simulink model "ROVSim_dp"  (R2022b)
settings: Solver=ode4  StartTime=0.0  StopTime=120  FixedStep=0.05  RelTol=1e-3
InitFcn:
  | initModelParam;
StopFcn:
  | %plotCoupled3DTrack;
libraries: slpidlib x9
settings Model: SimulationMode=accelerator  Creator=53549  LastModifiedBy=18144
settings SolverCC: AlgebraicLoopSolver=TrustRegion
settings DataIOCC: ReturnWorkspaceOutputs=off
settings DebuggingCC: UnconnectedInputMsg=warning  UnconnectedOutputMsg=warning  UnconnectedLineMsg=warning  SFMachineParentedDataDiag=warning  ArithmeticOperatorsInVariantConditions=warning
settings ModelReferenceCC: EnableRefExpFcnMdlSchedulingChecks=on
settings SFSimCC: SimUseLocalCustomCode=off  CustomCodeUndefinedFunction=UseInterfaceOnly
settings RTWCC: RTWUseLocalCustomCode=off  DLArmComputeVersion=19.05
settings CodeAppCC: StateflowObjectComments=on

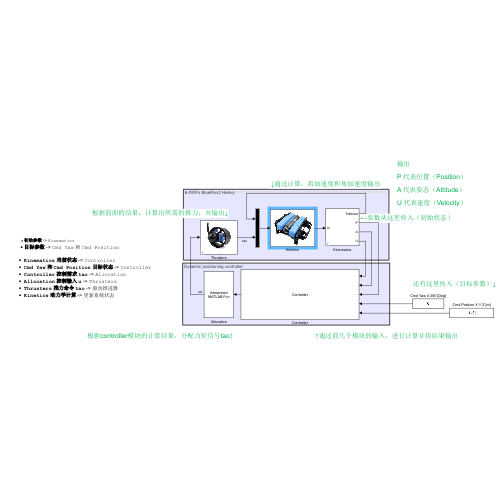
[thumbnail: Simulink's stored preview of the top-level diagram]
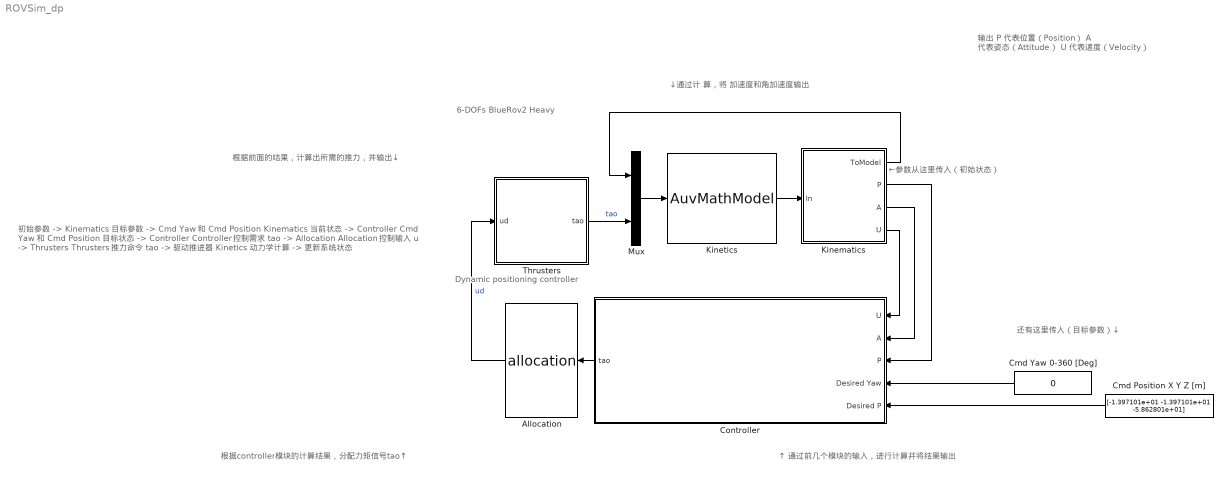
== system ROVSim_dp ==
  note: 初始参数 -> Kinematics
      | 目标参数 -> Cmd Yaw 和 Cmd Position
      |
      | Kinematics 当前状态 -> Controller
      | Cmd Yaw 和 Cmd Position 目标状态 -> Controller
      | Controller 控制需求 tao -> Allocation
      | Allocation 控制输入 u -> Thrusters
      | Thrusters 推力命令 tao -> 驱动推进器
      | Kinetics 动力学计算 -> 更新系统状态
  note: 输出
      | P 代表位置（Position）
      | A 代表姿态（Attitude）
      | U 代表速度（Velocity）
  note: ←参数从这里传入（初始状态）
  note: Dynamic positioning controller
  note: 6-DOFs BlueRov2 Heavy
  note: 还有这里传入（目标参数）↓
  note: ↑ 通过前几个模块的输入，进行计算并将结果输出
  note: 根据controller模块的计算结果，分配力矩信号tao↑
  note: 根据前面的结果，计算出所需的推力，并输出↓
  note: ↓通过计 算，将 加速度和角加速度输出
  Allocation : MATLABFcn  Description=|  MATLABFcn=allocation  OutputDimensions=8  OutputSignalType=real
      | Allocation模块功能:
      |  - 接收控制力和力矩信号tao
      |  - 使用控制分配矩阵Kni和转换矩阵Tni
      |  - 通过矩阵乘法将控制需求分配到各个推进器或执行机构
      |  - 输出控制输入u，用于驱动推进器或其他执行机构
  Cmd Position X Y Z [m] : Constant  Value=[-1.397101e+01 -1.397101e+01 -5.862801e+01]
  Cmd Yaw 0-360 [Deg] : Constant  Value=0
  Controller : Subsystem  Description=|
      | Controller模块功能:
      |  - 接收当前的位置信号P和姿态信号A
      |  - 接收期望的目标位置Desired P和艏向Desired Yaw
      |  - 通过PID控制器计算各个方向和角度的控制力和力矩信号
      |  - 输出控制信号tao_X、tao_Y、tao_Z、tao_K、tao_M和tao_N
      |  - 这些控制信号用于驱动船只的推进器或其他执行机构
      |  - 实现船只的精确运动和姿态控制
      mask Display: disp('Controller')
  Kinematics : Subsystem  Description=|  mask{x0=0.00, y0=0.00, z0=-40.00, pitch0=0, yaw0=138.72, u0=0, flowDir=45, flowVel=0.2}
      | 模块结构分析
      | 输入信号：
      | 包括线速度（u, v, w）和角速度（p, q, r）的信号，这些信号来自于动力学模块或其他部分。
      | 积分运算：
      | 通过积分角速度得到姿态角度，通过积分线速度得到位置坐标。
      | 输出信号：
      | 输出位置（P）、姿态（A）和速度（U），这些信号被其他模块使用，例如控制器、导航系统等。
      mask prompts: x0 "Initiral x"; y0 "Initiral y"; z0 "Initiral z"; pitch0 "Initial pitch [Deg]"; yaw0 "Initial yaw [Deg]"; u0 "Initial velocity [m/s]"; flowDir "Flow direction [Deg]"; flowVel "Flow velocity [m/s]"
      mask DialogControl DescGroupVar Prompt: Kinematics
      mask DialogControl DescTextVar Prompt: Set kinematics information: AMV initial state, flow interference, etc
      mask DialogControl ParameterGroupVar Prompt: Initial state
      mask DialogControl Container3 Prompt: Flow
  Kinetics : MATLABFcn  Description=|  MATLABFcn=AuvMathModel  OutputDimensions=6  OutputSignalType=real
      | Kinetics模块功能:
      |  - 接收当前的速度、角速度、姿态角度和控制力矩输入
      |  - 计算刚体和附加质量的科里奥利力和离心力矩阵
      |  - 计算流体阻尼力矩和重力浮力矩阵
      |  - 结合上述力矩计算总的作用力和力矩
      |  - 通过总质量矩阵的逆矩阵计算线加速度和角加速度输出
      |  
      |  输入参数:
      |  - u, v, w: 线速度分量
      |  - p, q, r: 角速度分量
      |  - phi, theta: 姿态角度
      |  - tao: 控制力和力矩
      | 
      |  输出参数:
      |  - dotu: 线加速度在x方向的分量，表示前进/后退方向的加速度变化
      |  - dotv: 线加速度在y方向的分量，表示左右侧移方向的加速度变化
      |  - dotw: 线加速度在z方向的分量，表示上下移动方向的加速度变化
      |  - dotp: 角加速度在p方向的分量，表示滚转方向的角加速度变化
      |  - dotq: 角加速度在q方向的分量，表示俯仰方向的角加速度变化
      |  - dotr: 角加速度在r方向的分量，表示偏航方向的角加速度变化
      mask Display: image('E:\个人文件\文件\大学\课题研究\水下机器人\仿真环境搭建\ROV\cover\blueRov.jpg'); % 使用工具条上的 "编辑图像" 进行更改。
  Mux : Mux  Inputs=2
  Thrusters : Subsystem  mask{dead_up=0.02, dead_low=-0.02, asym_gain=0.85}
      mask prompts: dead_up "Dead Zone Up Boundary [0, 1]"; dead_low "Dead Zone Low Boundary [-1, 0]"; asym_gain "Asymmetric Gain [0, 1]"
      mask DialogControl DescGroupVar Prompt: Thrusters model
      mask DialogControl DescTextVar Prompt: Thruster dead zone characteristic: When the input is near 0, the thruster does not rotate. Asymmetric characteristics of thrusters: With the same input, the thrust generated by reverse rotation of thrusters is less than that of forward rotation.
      mask Display: image('E:\个人文件\文件\大学\课题研究\水下机器人\仿真环境搭建\ROV\cover\thruster.jfif'); % 使用工具条上的 "编辑图像" 进行更改。
  wires:
  Kinetics/1 -> Kinematics/1(In)
  Mux/1 -> Kinetics/1
  Kinematics/1(ToModel) -> Mux/1
  Kinematics/2(P) -> Controller/3(P)
  Thrusters/1(tao) -> Mux/2  "tao"
  Cmd Yaw 0-360 [Deg]/1 -> Controller/4(Desired Yaw)
  Cmd Position X Y Z [m]/1 -> Controller/5(Desired P)
  Controller/1(tao) -> Allocation/1
  Allocation/1 -> Thrusters/1(ud)  "ud"
  Kinematics/3(A) -> Controller/2(A)
  Kinematics/4(U) -> Controller/1(U)

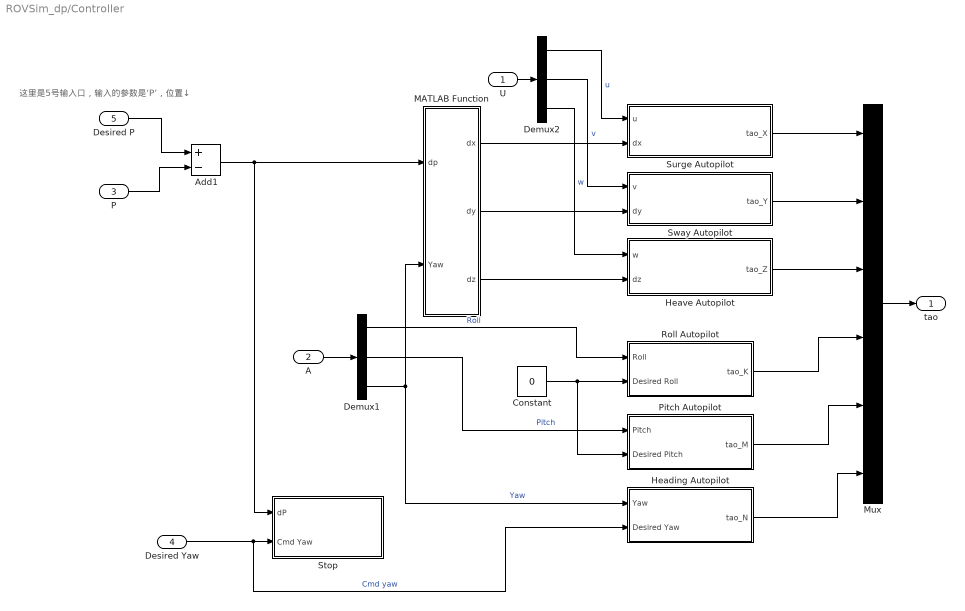
== system ROVSim_dp/Controller ==
  note: 这里是5号输入口，输入的参数是‘P’，位置↓
  U : Inport
  A : Inport  Port=2
  P : Inport  Port=3
  Desired Yaw : Inport  Port=4
  Desired P : Inport  Port=5
  Add1 : Sum  Inputs=+-
  Constant : Constant  Value=0
  Demux1 : Demux  Outputs=3
  Demux2 : Demux  Outputs=3
  Heading Autopilot : Subsystem  mask{kp=0.2, ki=0, kd=0.2}
      mask DialogControl DescGroupVar Prompt: Heading Autopilot
      mask DialogControl DescTextVar Prompt: 设置PID增益。
      mask DialogControl ParameterGroupVar Prompt: PID Parameter
  Heave Autopilot : Subsystem
  MATLAB Function : MATLAB Function  TreatAsAtomicUnit=on
  Mux : Mux  Inputs=6
  Pitch Autopilot : Subsystem  mask{kp=5, ki=0, kd=0}
      mask DialogControl DescGroupVar Prompt: Heading Autopilot
      mask DialogControl DescTextVar Prompt: 设置PID增益。
      mask DialogControl ParameterGroupVar Prompt: PID Parameter
  Roll Autopilot : Subsystem  mask{kp=5, ki=0, kd=0}
      mask DialogControl DescGroupVar Prompt: Heading Autopilot
      mask DialogControl DescTextVar Prompt: 设置PID增益。
      mask DialogControl ParameterGroupVar Prompt: PID Parameter
  Stop : Subsystem
  Surge Autopilot : Subsystem
  Sway Autopilot : Subsystem
  tao : Outport
  wires:
  Demux1/3 -> Heading Autopilot/1(Yaw), MATLAB Function/2(Yaw)  "Yaw"
  Constant/1 -> Pitch Autopilot/2(Desired Pitch), Roll Autopilot/2(Desired Roll)
  Demux1/2 -> Pitch Autopilot/1(Pitch)  "Pitch"
  A/1 -> Demux1/1
  Desired P/1 -> Add1/1
  Add1/1 -> MATLAB Function/1(dp), Stop/1(dP)
  P/1 -> Add1/2
  Roll Autopilot/1(tao_K) -> Mux/4
  Pitch Autopilot/1(tao_M) -> Mux/5
  Heading Autopilot/1(tao_N) -> Mux/6
  Mux/1 -> tao/1
  Demux1/1 -> Roll Autopilot/1(Roll)  "Roll"
  U/1 -> Demux2/1
  Demux2/1 -> Surge Autopilot/1(u)  "u"
  MATLAB Function/1(dx) -> Surge Autopilot/2(dx)
  Surge Autopilot/1(tao_X) -> Mux/1
  Demux2/2 -> Sway Autopilot/1(v)  "v"
  MATLAB Function/2(dy) -> Sway Autopilot/2(dy)
  Sway Autopilot/1(tao_Y) -> Mux/2
  Demux2/3 -> Heave Autopilot/1(w)  "w"
  MATLAB Function/3(dz) -> Heave Autopilot/2(dz)
  Heave Autopilot/1(tao_Z) -> Mux/3
  Desired Yaw/1 -> Heading Autopilot/2(Desired Yaw), Stop/2(Cmd Yaw)  "Cmd yaw"

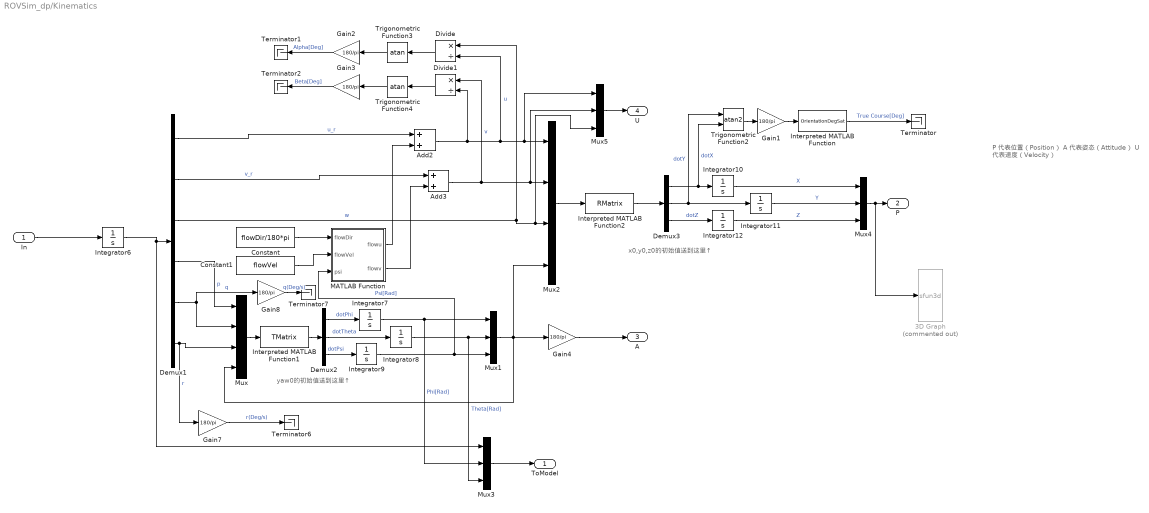
== system ROVSim_dp/Kinematics ==
  note: x0,y0,z0的初始值送到这里↑
  note: yaw0的初始值送到这里↑
  note: P 代表位置（Position）
      | A 代表姿态（Attitude）
      | U 代表速度（Velocity）
  In : Inport
  3D Graph : S-Function  Commented=on  LoadFcn=if exist('sfun3d','file'), sfun3d([],[],[],'LoadBlock'); end  FunctionName=sfun3d  Parameters=ax,T,np,cp,gd,ls,mk,mx,hd,tb  SFunctionDeploymentMode=off  EnableBusSupport=off  mask(3D Graph){np=1, ax=[-15 15 -15 15 -5 20], mx=1e4, T=0.1, cp=[3 2 1], gd=on, hd=on, tb=off, ls=-, mk=none}
      mask prompts: np "Number of moving points (lines)"; ax "Range: [xmin xmax  ymin ymax zmin zmax]"; mx "Max number of points in each line"; T "Sampling Time"; cp "Camera position (use [0 0 1] for 2D XY view)"; gd "Grid (on|off)"; hd "HeadMarkers (on|off)"; tb "Toolbar (on|off)"; ls "LineStyle"; mk "LineMarker"
      mask help:
      | This block plots the position of several points in the XYZ space. The input contains the coordinates of all the points (x1,y1,z1,x2,y2,z2,...).
      | The number of moving points (lines), the XYZ ranges, sampling time, camera position, and grid (among other things) can be set as mask parameters.
      settings: CopyFcn=if exist('sfun3d','file'), sfun3d([],[],[],'CopyBlock'); end  DeleteFcn=if exist('sfun3d','file'), sfun3d([],[],[],'DeleteBlock'); end  NameChangeFcn=if exist('sfun3d','file'), sfun3d([],[],[],'NameChange'); end
      mask Help:
      | This block plots the position of several points in the XYZ space. The input contains the coordinates of all the points (x1,y1,z1,x2,y2,z2,...).
      | The number of moving points (lines), the XYZ ranges, sampling time, camera position, and grid (among other things) can be set as mask parameters.
      mask TypeOptions ls: - | -- | : | -. | none
      mask TypeOptions mk: none | . | + | o | * | x | square | diamond | v | ^ | > | < | pentagram | hexagram
      mask Display: plot([.05 .95 .95 .05 .05],[.45 .45 .95 .95 .45], 0.5+cos(0:0.1:2*pi)*0.3,0.7+sin(0:0.1:2*pi)*0.2)
  Add2 : Sum
  Add3 : Sum
  Constant : Constant  Value=flowDir/180*pi
  Constant1 : Constant  Value=flowVel
  Demux1 : Demux  Outputs=6
  Demux2 : Demux  Outputs=3
  Demux3 : Demux  Outputs=3
  Divide : Product  Inputs=*/
  Divide1 : Product  Inputs=*/
  Gain{1..4,7..8} (6 alike) : Gain  Gain=180/pi
  Integrator10 : Integrator  InitialCondition=x0
  Integrator11 : Integrator  InitialCondition=y0
  Integrator12 : Integrator  InitialCondition=z0
  Integrator6 : Integrator  InitialCondition=[u0; 0; 0; 0; 0; 0]
  Integrator7 : Integrator
  Integrator8 : Integrator
  Integrator9 : Integrator  InitialCondition=yaw0*pi/180  WrapState=on  WrappedStateUpperValue=6.2832  WrappedStateLowerValue=0
  Interpreted MATLAB Function : MATLABFcn  MATLABFcn=OrientationDegSat
  Interpreted MATLAB Function1 : MATLABFcn  MATLABFcn=TMatrix  OutputDimensions=3
  Interpreted MATLAB Function2 : MATLABFcn  MATLABFcn=RMatrix  OutputDimensions=3
  MATLAB Function : MATLAB Function  TreatAsAtomicUnit=on
  Mux : Mux
  Mux{1,3..5} (4 alike) : Mux  Inputs=3
  Mux2 : Mux
  Terminator{,1..2,6..7} (5 alike) : Terminator
  Trigonometric Function2 : Trigonometry  Operator=atan2
  Trigonometric Function3 : Trigonometry  Operator=atan
  Trigonometric Function4 : Trigonometry  Operator=atan
  ToModel : Outport
  P : Outport  Port=2
  A : Outport  Port=3
  U : Outport  Port=4
  wires:
  Constant/1 -> MATLAB Function/1(flowDir)
  Constant1/1 -> MATLAB Function/2(flowVel)
  Integrator6/1 -> Mux3/1, Demux1/1
  Demux1/4 -> Mux/1  "p"
  Demux1/5 -> Gain8/1, Mux/2  "q"
  Demux1/6 -> Gain7/1, Mux/3  "r"
  Mux/1 -> Interpreted MATLAB Function1/1
  Interpreted MATLAB Function1/1 -> Demux2/1
  Demux2/1 -> Integrator7/1  "dotPhi"
  Demux2/2 -> Integrator8/1  "dotTheta"
  Demux2/3 -> Integrator9/1  "dotPsi"
  Integrator9/1 -> MATLAB Function/3(psi), Mux1/3  "Psi[Rad]"
  Integrator7/1 -> Mux1/1, Mux3/2  "Phi[Rad]"
  Integrator8/1 -> Mux3/3, Mux1/2  "Theta[Rad]"
  Mux1/1 -> Gain4/1, Mux/4, Mux2/4
  Demux1/1 -> Add2/1  "u_r"
  Demux1/2 -> Add3/1  "v_r"
  Demux1/3 -> Mux5/3, Mux2/3, Divide/1  "w"
  Mux2/1 -> Interpreted MATLAB Function2/1
  Interpreted MATLAB Function2/1 -> Demux3/1
  Demux3/1 -> Trigonometric Function2/2, Integrator10/1  "dotX"
  Demux3/2 -> Trigonometric Function2/1, Integrator11/1  "dotY"
  Demux3/3 -> Integrator12/1  "dotZ"
  Integrator10/1 -> Mux4/1  "X"
  Integrator11/1 -> Mux4/2  "Y"
  Integrator12/1 -> Mux4/3  "Z"
  Gain2/1 -> Terminator1/1  "Alpha[Deg]"
  Trigonometric Function3/1 -> Gain2/1
  Divide/1 -> Trigonometric Function3/1
  Divide1/1 -> Trigonometric Function4/1
  Trigonometric Function4/1 -> Gain3/1
  Gain3/1 -> Terminator2/1  "Beta[Deg]"
  Gain1/1 -> Interpreted MATLAB Function/1
  Interpreted MATLAB Function/1 -> Terminator/1  "True Course[Deg]"
  Trigonometric Function2/1 -> Gain1/1
  Add2/1 -> Divide1/2, Divide/2, Mux5/1, Mux2/1  "u"
  Add3/1 -> Mux5/2, Mux2/2, Divide1/1  "v"
  MATLAB Function/1(flowu) -> Add2/2
  MATLAB Function/2(flowv) -> Add3/2
  Mux3/1 -> ToModel/1
  Mux4/1 -> 3D Graph/1, P/1
  In/1 -> Integrator6/1
  Gain7/1 -> Terminator6/1  "r(Deg/s)"
  Gain8/1 -> Terminator7/1  "q(Deg/s)"
  Gain4/1 -> A/1
  Mux5/1 -> U/1

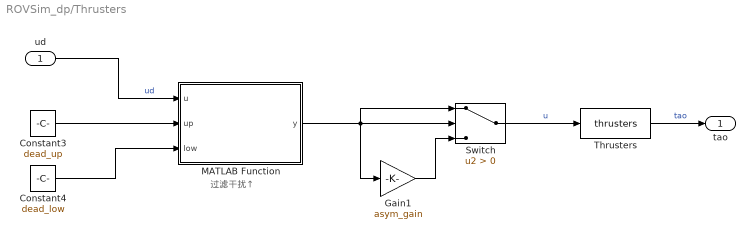
== system ROVSim_dp/Thrusters ==
  note: 过滤干扰↑
  ud : Inport
  Constant3 : Constant  Value=dead_up
  Constant4 : Constant  Value=dead_low
  Gain1 : Gain  Gain=asym_gain
  MATLAB Function : MATLAB Function  TreatAsAtomicUnit=on
  Switch : Switch  Criteria=u2 > Threshold  SaturateOnIntegerOverflow=off  InputSameDT=off
  Thrusters : MATLABFcn  MATLABFcn=thrusters  OutputDimensions=6  OutputSignalType=real
  tao : Outport
  wires:
  Thrusters/1 -> tao/1  "tao"
  ud/1 -> MATLAB Function/1(u)  "ud"
  Gain1/1 -> Switch/3
  MATLAB Function/1(y) -> Switch/1, Gain1/1, Switch/2
  Constant4/1 -> MATLAB Function/3(low)
  Switch/1 -> Thrusters/1  "u"
  Constant3/1 -> MATLAB Function/2(up)

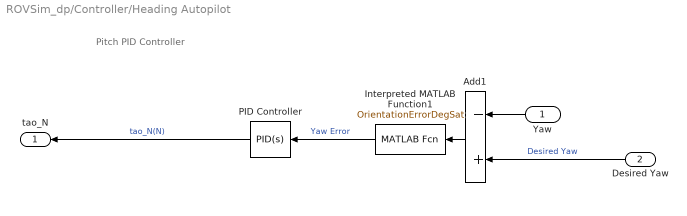
== system ROVSim_dp/Controller/Heading Autopilot ==
  note: Pitch PID Controller
  Yaw : Inport
  Desired Yaw : Inport  Port=2
  Add1 : Sum  Inputs=-+
  Interpreted MATLAB Function1 : MATLABFcn  MATLABFcn=OrientationErrorDegSat  OutputDimensions=1
  PID Controller : slpidlib/PID Controller  Controller=PID  Form=Parallel  TimeDomain=Continuous-time  UseExternalTs=off  SampleTime=-1  IntegratorMethod=Forward Euler  FilterMethod=Forward Euler  ControllerParametersSource=internal  P=kp  I=ki  UseKiTs=off  D=kd  N=10  UseFilter=on  TunerSelectOption=Transfer Function Based (PID Tuner App)  InitialConditionSource=internal  InitialConditionForIntegrator=0  InitialConditionForFilter=0  DifferentiatorICPrevScaledInput=0  ExternalReset=none  TrackingMode=off  Kt=1  LimitOutput=on  SatLimitsSource=internal  UpperSaturationLimit=20  LowerSaturationLimit=-20  LinearizeAsGain=on  AntiWindupMode=none  Kb=1  LimitIntegrator=off  UpperIntegratorSaturationLimit=inf  LowerIntegratorSaturationLimit=-inf  POutMin=[]  POutMax=[]  IOutMin=[]  IOutMax=[]  DOutMin=[]  DOutMax=[]  NOutMin=[]  NOutMax=[]  SumOutMin=[]  SumOutMax=[]  SaturationOutMin=[]  SaturationOutMax=[]  PParamMin=[]  PParamMax=[]  IParamMin=[]  IParamMax=[]  DParamMin=[]  DParamMax=[]  NParamMin=[]  NParamMax=[]  KbParamMin=[]  KbParamMax=[]  KtParamMin=[]  KtParamMax=[]  KbOutMin=[]  KbOutMax=[]  KtOutMin=[]  KtOutMax=[]  IntegratorOutMin=[]  IntegratorOutMax=[]  FilterOutMin=[]  FilterOutMax=[]  SumI1OutMin=[]  SumI1OutMax=[]  SumI2OutMin=[]  SumI2OutMax=[]  SumI3OutMin=[]  SumI3OutMax=[]  SumI4OutMin=[]  SumI4OutMax=[]  SumDOutMin=[]  SumDOutMax=[]  DifferentiatorOutMin=[]  DifferentiatorOutMax=[]  FilterDiffOutCoefMin=[]  FilterDiffOutCoefMax=[]  ReciprocalOutMin=[]  ReciprocalOutMax=[]  SumDenOutMin=[]  SumDenOutMax=[]  SumNumOutMin=[]  SumNumOutMax=[]  DivideOutMin=[]  DivideOutMax=[]  UdiffTsProdOutMin=[]  UdiffTsProdOutMax=[]  NTsProdOutMin=[]  NTsProdOutMax=[]  UintegralTsProdOutMin=[]  UintegralTsProdOutMax=[]  UngainTsProdOutMin=[]  UngainTsProdOutMax=[]  ClampingZeroOutDataTypeStr=Inherit: Inherit via back propagation  ClampingZeroOutMin=[]  ClampingZeroOutMax=[]  FilterDenConstantOutDataTypeStr=Inherit: Inherit via back propagation  FilterDenConstantOutMin=[]  FilterDenConstantOutMax=[]  PCopyOutDataTypeStr=Inherit: Inherit via back propagation  PCopyOutMin=[]  PCopyOutMax=[]  NCopyOutDataTypeStr=Inherit: Inherit via back propagation  NCopyOutMin=[]  NCopyOutMax=[]  IntegratorContinuousStateAttributes=''  IntegratorStateMustResolveToSignalObject=off  IntegratorRTWStateStorageClass=Auto  FilterContinuousStateAttributes=''  FilterStateMustResolveToSignalObject=off  FilterRTWStateStorageClass=Auto  ParallelPVariant=InternalParameters  IdealPVariant=Disabled  IVariant=InternalParameters  DVariant=InternalParameters  IntegratorVariant=Continuous  SatVariant=Enabled  AWVariant=Passthrough  PCopyVariant=Disabled  TRVariant=Disabled  FdbkBlocksVariant=Forward  IdealPFdbkVariant=Disabled  SatFdbkVariant=Disabled  DerivativeFilterVariant=ContFilter  NVariant=InternalParameters  NCopyVariant=Disabled  FilterICVariant=InternalICsFilter  IntegratorICVariant=InternalICs  ExternalResetVariant=Disabled  TRSumVariant=Passthrough  SumFdbkVariant=Disabled  SumVariant=Sum_PID  TsampFilterVariant=InternalTs  TsampNgainVariant=Passthrough  TsampIntegralVariant=Passthrough  ExternalSaturationOutDataTypeStr=Inherit: Same as second input
  tao_N : Outport
  wires:
  Yaw/1 -> Add1/1
  PID Controller/1 -> tao_N/1  "tao_N(N)"
  Add1/1 -> Interpreted MATLAB Function1/1
  Desired Yaw/1 -> Add1/2  "Desired Yaw"
  Interpreted MATLAB Function1/1 -> PID Controller/1  "Yaw Error"

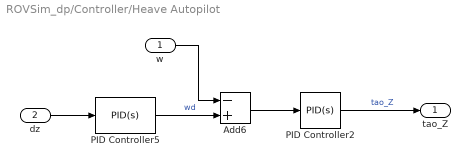
== system ROVSim_dp/Controller/Heave Autopilot ==
  w : Inport
  dz : Inport  Port=2
  Add6 : Sum  Inputs=-+
  PID Controller2 : slpidlib/PID Controller  Controller=PID  Form=Parallel  TimeDomain=Continuous-time  UseExternalTs=off  SampleTime=-1  IntegratorMethod=Forward Euler  FilterMethod=Forward Euler  ControllerParametersSource=internal  P=40  I=0.5  UseKiTs=off  D=0  N=100  UseFilter=on  TunerSelectOption=Transfer Function Based (PID Tuner App)  InitialConditionSource=internal  InitialConditionForIntegrator=0  InitialConditionForFilter=0  DifferentiatorICPrevScaledInput=0  ExternalReset=none  TrackingMode=off  Kt=1  LimitOutput=off  SatLimitsSource=internal  UpperSaturationLimit=inf  LowerSaturationLimit=-inf  LinearizeAsGain=on  AntiWindupMode=none  Kb=1  LimitIntegrator=off  UpperIntegratorSaturationLimit=inf  LowerIntegratorSaturationLimit=-inf  POutMin=[]  POutMax=[]  IOutMin=[]  IOutMax=[]  DOutMin=[]  DOutMax=[]  NOutMin=[]  NOutMax=[]  SumOutMin=[]  SumOutMax=[]  SaturationOutMin=[]  SaturationOutMax=[]  PParamMin=[]  PParamMax=[]  IParamMin=[]  IParamMax=[]  DParamMin=[]  DParamMax=[]  NParamMin=[]  NParamMax=[]  KbParamMin=[]  KbParamMax=[]  KtParamMin=[]  KtParamMax=[]  KbOutMin=[]  KbOutMax=[]  KtOutMin=[]  KtOutMax=[]  IntegratorOutMin=[]  IntegratorOutMax=[]  FilterOutMin=[]  FilterOutMax=[]  SumI1OutMin=[]  SumI1OutMax=[]  SumI2OutMin=[]  SumI2OutMax=[]  SumI3OutMin=[]  SumI3OutMax=[]  SumI4OutMin=[]  SumI4OutMax=[]  SumDOutMin=[]  SumDOutMax=[]  DifferentiatorOutMin=[]  DifferentiatorOutMax=[]  FilterDiffOutCoefMin=[]  FilterDiffOutCoefMax=[]  ReciprocalOutMin=[]  ReciprocalOutMax=[]  SumDenOutMin=[]  SumDenOutMax=[]  SumNumOutMin=[]  SumNumOutMax=[]  DivideOutMin=[]  DivideOutMax=[]  UdiffTsProdOutMin=[]  UdiffTsProdOutMax=[]  NTsProdOutMin=[]  NTsProdOutMax=[]  UintegralTsProdOutMin=[]  UintegralTsProdOutMax=[]  UngainTsProdOutMin=[]  UngainTsProdOutMax=[]  ClampingZeroOutDataTypeStr=Inherit: Inherit via back propagation  ClampingZeroOutMin=[]  ClampingZeroOutMax=[]  FilterDenConstantOutDataTypeStr=Inherit: Inherit via back propagation  FilterDenConstantOutMin=[]  FilterDenConstantOutMax=[]  PCopyOutDataTypeStr=Inherit: Inherit via back propagation  PCopyOutMin=[]  PCopyOutMax=[]  NCopyOutDataTypeStr=Inherit: Inherit via back propagation  NCopyOutMin=[]  NCopyOutMax=[]  IntegratorContinuousStateAttributes=''  IntegratorStateMustResolveToSignalObject=off  IntegratorRTWStateStorageClass=Auto  FilterContinuousStateAttributes=''  FilterStateMustResolveToSignalObject=off  FilterRTWStateStorageClass=Auto  ParallelPVariant=InternalParameters  IdealPVariant=Disabled  IVariant=InternalParameters  DVariant=InternalParameters  IntegratorVariant=Continuous  SatVariant=Disabled  AWVariant=Passthrough  PCopyVariant=Disabled  TRVariant=Disabled  FdbkBlocksVariant=Forward  IdealPFdbkVariant=Disabled  SatFdbkVariant=Disabled  DerivativeFilterVariant=ContFilter  NVariant=InternalParameters  NCopyVariant=Disabled  FilterICVariant=InternalICsFilter  IntegratorICVariant=InternalICs  ExternalResetVariant=Disabled  TRSumVariant=Passthrough  SumFdbkVariant=Disabled  SumVariant=Sum_PID  TsampFilterVariant=InternalTs  TsampNgainVariant=Passthrough  TsampIntegralVariant=Passthrough  ExternalSaturationOutDataTypeStr=Inherit: Same as second input
  PID Controller5 : slpidlib/PID Controller  Controller=PID  Form=Parallel  TimeDomain=Continuous-time  UseExternalTs=off  SampleTime=-1  IntegratorMethod=Forward Euler  FilterMethod=Forward Euler  ControllerParametersSource=internal  P=0.5  I=0  UseKiTs=off  D=0  N=100  UseFilter=on  TunerSelectOption=Transfer Function Based (PID Tuner App)  InitialConditionSource=internal  InitialConditionForIntegrator=0  InitialConditionForFilter=0  DifferentiatorICPrevScaledInput=0  ExternalReset=none  TrackingMode=off  Kt=1  LimitOutput=on  SatLimitsSource=internal  UpperSaturationLimit=1  LowerSaturationLimit=-1  LinearizeAsGain=on  AntiWindupMode=none  Kb=1  LimitIntegrator=off  UpperIntegratorSaturationLimit=inf  LowerIntegratorSaturationLimit=-inf  POutMin=[]  POutMax=[]  IOutMin=[]  IOutMax=[]  DOutMin=[]  DOutMax=[]  NOutMin=[]  NOutMax=[]  SumOutMin=[]  SumOutMax=[]  SaturationOutMin=[]  SaturationOutMax=[]  PParamMin=[]  PParamMax=[]  IParamMin=[]  IParamMax=[]  DParamMin=[]  DParamMax=[]  NParamMin=[]  NParamMax=[]  KbParamMin=[]  KbParamMax=[]  KtParamMin=[]  KtParamMax=[]  KbOutMin=[]  KbOutMax=[]  KtOutMin=[]  KtOutMax=[]  IntegratorOutMin=[]  IntegratorOutMax=[]  FilterOutMin=[]  FilterOutMax=[]  SumI1OutMin=[]  SumI1OutMax=[]  SumI2OutMin=[]  SumI2OutMax=[]  SumI3OutMin=[]  SumI3OutMax=[]  SumI4OutMin=[]  SumI4OutMax=[]  SumDOutMin=[]  SumDOutMax=[]  DifferentiatorOutMin=[]  DifferentiatorOutMax=[]  FilterDiffOutCoefMin=[]  FilterDiffOutCoefMax=[]  ReciprocalOutMin=[]  ReciprocalOutMax=[]  SumDenOutMin=[]  SumDenOutMax=[]  SumNumOutMin=[]  SumNumOutMax=[]  DivideOutMin=[]  DivideOutMax=[]  UdiffTsProdOutMin=[]  UdiffTsProdOutMax=[]  NTsProdOutMin=[]  NTsProdOutMax=[]  UintegralTsProdOutMin=[]  UintegralTsProdOutMax=[]  UngainTsProdOutMin=[]  UngainTsProdOutMax=[]  ClampingZeroOutDataTypeStr=Inherit: Inherit via back propagation  ClampingZeroOutMin=[]  ClampingZeroOutMax=[]  FilterDenConstantOutDataTypeStr=Inherit: Inherit via back propagation  FilterDenConstantOutMin=[]  FilterDenConstantOutMax=[]  PCopyOutDataTypeStr=Inherit: Inherit via back propagation  PCopyOutMin=[]  PCopyOutMax=[]  NCopyOutDataTypeStr=Inherit: Inherit via back propagation  NCopyOutMin=[]  NCopyOutMax=[]  IntegratorContinuousStateAttributes=''  IntegratorStateMustResolveToSignalObject=off  IntegratorRTWStateStorageClass=Auto  FilterContinuousStateAttributes=''  FilterStateMustResolveToSignalObject=off  FilterRTWStateStorageClass=Auto  ParallelPVariant=InternalParameters  IdealPVariant=Disabled  IVariant=InternalParameters  DVariant=InternalParameters  IntegratorVariant=Continuous  SatVariant=Enabled  AWVariant=Passthrough  PCopyVariant=Disabled  TRVariant=Disabled  FdbkBlocksVariant=Forward  IdealPFdbkVariant=Disabled  SatFdbkVariant=Disabled  DerivativeFilterVariant=ContFilter  NVariant=InternalParameters  NCopyVariant=Disabled  FilterICVariant=InternalICsFilter  IntegratorICVariant=InternalICs  ExternalResetVariant=Disabled  TRSumVariant=Passthrough  SumFdbkVariant=Disabled  SumVariant=Sum_PID  TsampFilterVariant=InternalTs  TsampNgainVariant=Passthrough  TsampIntegralVariant=Passthrough  ExternalSaturationOutDataTypeStr=Inherit: Same as second input
  tao_Z : Outport
  wires:
  Add6/1 -> PID Controller2/1
  PID Controller5/1 -> Add6/2  "wd"
  dz/1 -> PID Controller5/1
  PID Controller2/1 -> tao_Z/1  "tao_Z"
  w/1 -> Add6/1

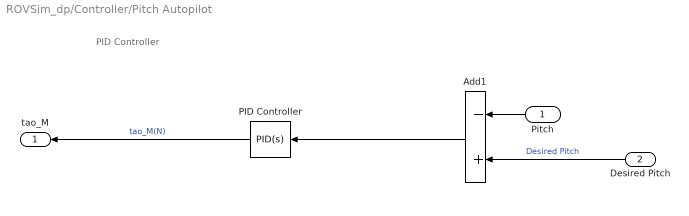
== system ROVSim_dp/Controller/Pitch Autopilot ==
  note: PID Controller
  Pitch : Inport
  Desired Pitch : Inport  Port=2
  Add1 : Sum  Inputs=-+
  PID Controller : slpidlib/PID Controller  Controller=PID  Form=Parallel  TimeDomain=Continuous-time  UseExternalTs=off  SampleTime=-1  IntegratorMethod=Forward Euler  FilterMethod=Forward Euler  ControllerParametersSource=internal  P=kp  I=ki  UseKiTs=off  D=kd  N=10  UseFilter=on  TunerSelectOption=Transfer Function Based (PID Tuner App)  InitialConditionSource=internal  InitialConditionForIntegrator=0  InitialConditionForFilter=0  DifferentiatorICPrevScaledInput=0  ExternalReset=none  TrackingMode=off  Kt=1  LimitOutput=on  SatLimitsSource=internal  UpperSaturationLimit=20  LowerSaturationLimit=-20  LinearizeAsGain=on  AntiWindupMode=none  Kb=1  LimitIntegrator=off  UpperIntegratorSaturationLimit=inf  LowerIntegratorSaturationLimit=-inf  POutMin=[]  POutMax=[]  IOutMin=[]  IOutMax=[]  DOutMin=[]  DOutMax=[]  NOutMin=[]  NOutMax=[]  SumOutMin=[]  SumOutMax=[]  SaturationOutMin=[]  SaturationOutMax=[]  PParamMin=[]  PParamMax=[]  IParamMin=[]  IParamMax=[]  DParamMin=[]  DParamMax=[]  NParamMin=[]  NParamMax=[]  KbParamMin=[]  KbParamMax=[]  KtParamMin=[]  KtParamMax=[]  KbOutMin=[]  KbOutMax=[]  KtOutMin=[]  KtOutMax=[]  IntegratorOutMin=[]  IntegratorOutMax=[]  FilterOutMin=[]  FilterOutMax=[]  SumI1OutMin=[]  SumI1OutMax=[]  SumI2OutMin=[]  SumI2OutMax=[]  SumI3OutMin=[]  SumI3OutMax=[]  SumI4OutMin=[]  SumI4OutMax=[]  SumDOutMin=[]  SumDOutMax=[]  DifferentiatorOutMin=[]  DifferentiatorOutMax=[]  FilterDiffOutCoefMin=[]  FilterDiffOutCoefMax=[]  ReciprocalOutMin=[]  ReciprocalOutMax=[]  SumDenOutMin=[]  SumDenOutMax=[]  SumNumOutMin=[]  SumNumOutMax=[]  DivideOutMin=[]  DivideOutMax=[]  UdiffTsProdOutMin=[]  UdiffTsProdOutMax=[]  NTsProdOutMin=[]  NTsProdOutMax=[]  UintegralTsProdOutMin=[]  UintegralTsProdOutMax=[]  UngainTsProdOutMin=[]  UngainTsProdOutMax=[]  ClampingZeroOutDataTypeStr=Inherit: Inherit via back propagation  ClampingZeroOutMin=[]  ClampingZeroOutMax=[]  FilterDenConstantOutDataTypeStr=Inherit: Inherit via back propagation  FilterDenConstantOutMin=[]  FilterDenConstantOutMax=[]  PCopyOutDataTypeStr=Inherit: Inherit via back propagation  PCopyOutMin=[]  PCopyOutMax=[]  NCopyOutDataTypeStr=Inherit: Inherit via back propagation  NCopyOutMin=[]  NCopyOutMax=[]  IntegratorContinuousStateAttributes=''  IntegratorStateMustResolveToSignalObject=off  IntegratorRTWStateStorageClass=Auto  FilterContinuousStateAttributes=''  FilterStateMustResolveToSignalObject=off  FilterRTWStateStorageClass=Auto  ParallelPVariant=InternalParameters  IdealPVariant=Disabled  IVariant=InternalParameters  DVariant=InternalParameters  IntegratorVariant=Continuous  SatVariant=Enabled  AWVariant=Passthrough  PCopyVariant=Disabled  TRVariant=Disabled  FdbkBlocksVariant=Forward  IdealPFdbkVariant=Disabled  SatFdbkVariant=Disabled  DerivativeFilterVariant=ContFilter  NVariant=InternalParameters  NCopyVariant=Disabled  FilterICVariant=InternalICsFilter  IntegratorICVariant=InternalICs  ExternalResetVariant=Disabled  TRSumVariant=Passthrough  SumFdbkVariant=Disabled  SumVariant=Sum_PID  TsampFilterVariant=InternalTs  TsampNgainVariant=Passthrough  TsampIntegralVariant=Passthrough  ExternalSaturationOutDataTypeStr=Inherit: Same as second input
  tao_M : Outport
  wires:
  Add1/1 -> PID Controller/1
  Desired Pitch/1 -> Add1/2  "Desired Pitch"
  PID Controller/1 -> tao_M/1  "tao_M(N)"
  Pitch/1 -> Add1/1

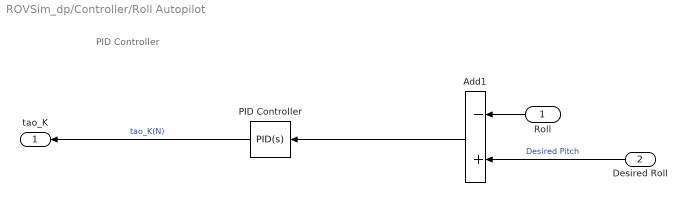
== system ROVSim_dp/Controller/Roll Autopilot ==
  note: PID Controller
  Roll : Inport
  Desired Roll : Inport  Port=2
  Add1 : Sum  Inputs=-+
  PID Controller : slpidlib/PID Controller  Controller=PID  Form=Parallel  TimeDomain=Continuous-time  UseExternalTs=off  SampleTime=-1  IntegratorMethod=Forward Euler  FilterMethod=Forward Euler  ControllerParametersSource=internal  P=kp  I=ki  UseKiTs=off  D=kd  N=10  UseFilter=on  TunerSelectOption=Transfer Function Based (PID Tuner App)  InitialConditionSource=internal  InitialConditionForIntegrator=0  InitialConditionForFilter=0  DifferentiatorICPrevScaledInput=0  ExternalReset=none  TrackingMode=off  Kt=1  LimitOutput=on  SatLimitsSource=internal  UpperSaturationLimit=20  LowerSaturationLimit=-20  LinearizeAsGain=on  AntiWindupMode=none  Kb=1  LimitIntegrator=off  UpperIntegratorSaturationLimit=inf  LowerIntegratorSaturationLimit=-inf  POutMin=[]  POutMax=[]  IOutMin=[]  IOutMax=[]  DOutMin=[]  DOutMax=[]  NOutMin=[]  NOutMax=[]  SumOutMin=[]  SumOutMax=[]  SaturationOutMin=[]  SaturationOutMax=[]  PParamMin=[]  PParamMax=[]  IParamMin=[]  IParamMax=[]  DParamMin=[]  DParamMax=[]  NParamMin=[]  NParamMax=[]  KbParamMin=[]  KbParamMax=[]  KtParamMin=[]  KtParamMax=[]  KbOutMin=[]  KbOutMax=[]  KtOutMin=[]  KtOutMax=[]  IntegratorOutMin=[]  IntegratorOutMax=[]  FilterOutMin=[]  FilterOutMax=[]  SumI1OutMin=[]  SumI1OutMax=[]  SumI2OutMin=[]  SumI2OutMax=[]  SumI3OutMin=[]  SumI3OutMax=[]  SumI4OutMin=[]  SumI4OutMax=[]  SumDOutMin=[]  SumDOutMax=[]  DifferentiatorOutMin=[]  DifferentiatorOutMax=[]  FilterDiffOutCoefMin=[]  FilterDiffOutCoefMax=[]  ReciprocalOutMin=[]  ReciprocalOutMax=[]  SumDenOutMin=[]  SumDenOutMax=[]  SumNumOutMin=[]  SumNumOutMax=[]  DivideOutMin=[]  DivideOutMax=[]  UdiffTsProdOutMin=[]  UdiffTsProdOutMax=[]  NTsProdOutMin=[]  NTsProdOutMax=[]  UintegralTsProdOutMin=[]  UintegralTsProdOutMax=[]  UngainTsProdOutMin=[]  UngainTsProdOutMax=[]  ClampingZeroOutDataTypeStr=Inherit: Inherit via back propagation  ClampingZeroOutMin=[]  ClampingZeroOutMax=[]  FilterDenConstantOutDataTypeStr=Inherit: Inherit via back propagation  FilterDenConstantOutMin=[]  FilterDenConstantOutMax=[]  PCopyOutDataTypeStr=Inherit: Inherit via back propagation  PCopyOutMin=[]  PCopyOutMax=[]  NCopyOutDataTypeStr=Inherit: Inherit via back propagation  NCopyOutMin=[]  NCopyOutMax=[]  IntegratorContinuousStateAttributes=''  IntegratorStateMustResolveToSignalObject=off  IntegratorRTWStateStorageClass=Auto  FilterContinuousStateAttributes=''  FilterStateMustResolveToSignalObject=off  FilterRTWStateStorageClass=Auto  ParallelPVariant=InternalParameters  IdealPVariant=Disabled  IVariant=InternalParameters  DVariant=InternalParameters  IntegratorVariant=Continuous  SatVariant=Enabled  AWVariant=Passthrough  PCopyVariant=Disabled  TRVariant=Disabled  FdbkBlocksVariant=Forward  IdealPFdbkVariant=Disabled  SatFdbkVariant=Disabled  DerivativeFilterVariant=ContFilter  NVariant=InternalParameters  NCopyVariant=Disabled  FilterICVariant=InternalICsFilter  IntegratorICVariant=InternalICs  ExternalResetVariant=Disabled  TRSumVariant=Passthrough  SumFdbkVariant=Disabled  SumVariant=Sum_PID  TsampFilterVariant=InternalTs  TsampNgainVariant=Passthrough  TsampIntegralVariant=Passthrough  ExternalSaturationOutDataTypeStr=Inherit: Same as second input
  tao_K : Outport
  wires:
  Roll/1 -> Add1/1
  PID Controller/1 -> tao_K/1  "tao_K(N)"
  Desired Roll/1 -> Add1/2  "Desired Pitch"
  Add1/1 -> PID Controller/1

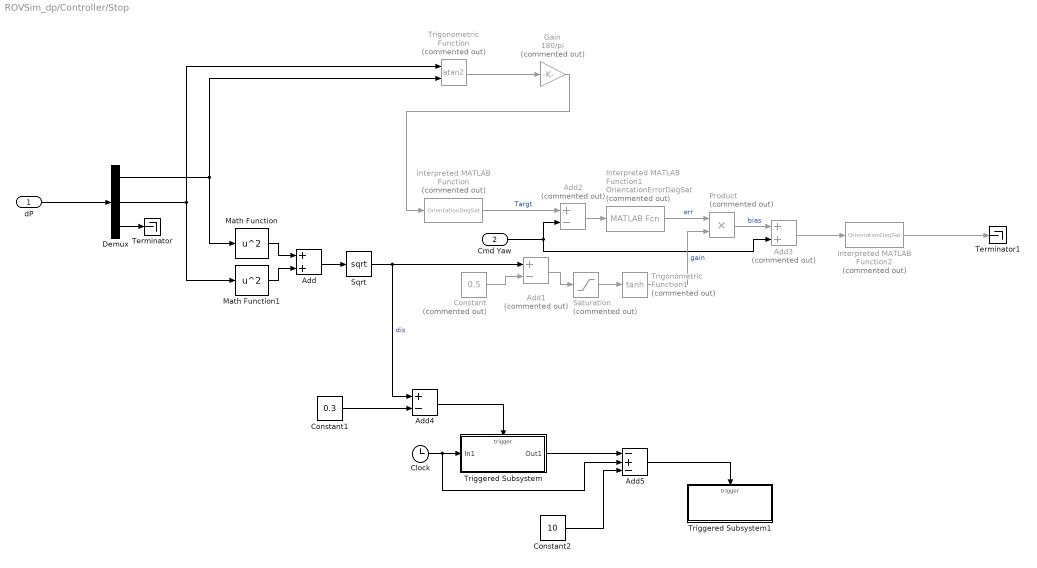
== system ROVSim_dp/Controller/Stop ==
  dP : Inport
  Cmd Yaw : Inport  Port=2
  Add : Sum
  Add1 : Sum  Commented=on  Inputs=+-
  Add2 : Sum  Commented=on  Inputs=+-
  Add3 : Sum  Commented=on
  Add4 : Sum  Inputs=+-
  Add5 : Sum  Inputs=-+-
  Clock : Clock
  Constant : Constant  Commented=on  Value=0.5
  Constant1 : Constant  Value=0.3
  Constant2 : Constant  Value=10
  Demux : Demux  Outputs=3
  Gain : Gain  Commented=on  Gain=180/pi
  Interpreted MATLAB Function : MATLABFcn  Commented=on  MATLABFcn=OrientationDegSat  OutputDimensions=1
  Interpreted MATLAB Function1 : MATLABFcn  Commented=on  MATLABFcn=OrientationErrorDegSat  OutputDimensions=1
  Interpreted MATLAB Function2 : MATLABFcn  Commented=on  MATLABFcn=OrientationDegSat  OutputDimensions=1
  Math Function : Math  Operator=square
  Math Function1 : Math  Operator=square
  Product : Product  Commented=on
  Saturation : Saturate  Commented=on  UpperLimit=inf  LowerLimit=0
  Sqrt : Sqrt
  Terminator : Terminator
  Terminator1 : Terminator
  Triggered Subsystem : Subsystem  TreatAsAtomicUnit=on
  Triggered Subsystem1 : Subsystem  TreatAsAtomicUnit=on
  Trigonometric Function : Trigonometry  Commented=on  Operator=atan2
  Trigonometric Function1 : Trigonometry  Commented=on  Operator=tanh
  wires:
  Math Function/1 -> Add/1
  Product/1 -> Add3/1  "bias"
  Interpreted MATLAB Function/1 -> Add2/1  "Targt"
  Cmd Yaw/1 -> Add2/2, Add3/2
  dP/1 -> Demux/1
  Gain/1 -> Interpreted MATLAB Function/1
  Demux/1 -> Math Function/1, Trigonometric Function/2
  Add3/1 -> Interpreted MATLAB Function2/1
  Interpreted MATLAB Function1/1 -> Product/1  "err"
  Demux/3 -> Terminator/1
  Trigonometric Function/1 -> Gain/1
  Demux/2 -> Math Function1/1, Trigonometric Function/1
  Add/1 -> Sqrt/1
  Sqrt/1 -> Add4/1, Add1/1  "dis"
  Add2/1 -> Interpreted MATLAB Function1/1
  Trigonometric Function1/1 -> Product/2  "gain"
  Math Function1/1 -> Add/2
  Interpreted MATLAB Function2/1 -> Terminator1/1
  Constant/1 -> Add1/2
  Add1/1 -> Saturation/1
  Saturation/1 -> Trigonometric Function1/1
  Constant1/1 -> Add4/2
  Add4/1 -> Triggered Subsystem/Trigger
  Clock/1 -> Add5/2, Triggered Subsystem/1(In1)
  Triggered Subsystem/1(Out1) -> Add5/1
  Add5/1 -> Triggered Subsystem1/Trigger
  Constant2/1 -> Add5/3

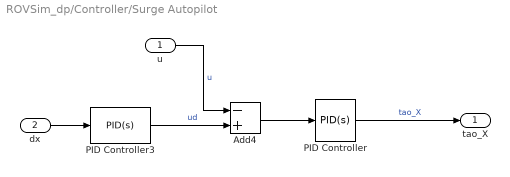
== system ROVSim_dp/Controller/Surge Autopilot ==
  u : Inport
  dx : Inport  Port=2
  Add4 : Sum  Inputs=-+
  PID Controller : slpidlib/PID Controller  Controller=PID  Form=Parallel  TimeDomain=Continuous-time  UseExternalTs=off  SampleTime=-1  IntegratorMethod=Forward Euler  FilterMethod=Forward Euler  ControllerParametersSource=internal  P=20  I=0  UseKiTs=off  D=0  N=100  UseFilter=on  TunerSelectOption=Transfer Function Based (PID Tuner App)  InitialConditionSource=internal  InitialConditionForIntegrator=0  InitialConditionForFilter=0  DifferentiatorICPrevScaledInput=0  ExternalReset=none  TrackingMode=off  Kt=1  LimitOutput=off  SatLimitsSource=internal  UpperSaturationLimit=inf  LowerSaturationLimit=-inf  LinearizeAsGain=on  AntiWindupMode=none  Kb=1  LimitIntegrator=off  UpperIntegratorSaturationLimit=inf  LowerIntegratorSaturationLimit=-inf  POutMin=[]  POutMax=[]  IOutMin=[]  IOutMax=[]  DOutMin=[]  DOutMax=[]  NOutMin=[]  NOutMax=[]  SumOutMin=[]  SumOutMax=[]  SaturationOutMin=[]  SaturationOutMax=[]  PParamMin=[]  PParamMax=[]  IParamMin=[]  IParamMax=[]  DParamMin=[]  DParamMax=[]  NParamMin=[]  NParamMax=[]  KbParamMin=[]  KbParamMax=[]  KtParamMin=[]  KtParamMax=[]  KbOutMin=[]  KbOutMax=[]  KtOutMin=[]  KtOutMax=[]  IntegratorOutMin=[]  IntegratorOutMax=[]  FilterOutMin=[]  FilterOutMax=[]  SumI1OutMin=[]  SumI1OutMax=[]  SumI2OutMin=[]  SumI2OutMax=[]  SumI3OutMin=[]  SumI3OutMax=[]  SumI4OutMin=[]  SumI4OutMax=[]  SumDOutMin=[]  SumDOutMax=[]  DifferentiatorOutMin=[]  DifferentiatorOutMax=[]  FilterDiffOutCoefMin=[]  FilterDiffOutCoefMax=[]  ReciprocalOutMin=[]  ReciprocalOutMax=[]  SumDenOutMin=[]  SumDenOutMax=[]  SumNumOutMin=[]  SumNumOutMax=[]  DivideOutMin=[]  DivideOutMax=[]  UdiffTsProdOutMin=[]  UdiffTsProdOutMax=[]  NTsProdOutMin=[]  NTsProdOutMax=[]  UintegralTsProdOutMin=[]  UintegralTsProdOutMax=[]  UngainTsProdOutMin=[]  UngainTsProdOutMax=[]  ClampingZeroOutDataTypeStr=Inherit: Inherit via back propagation  ClampingZeroOutMin=[]  ClampingZeroOutMax=[]  FilterDenConstantOutDataTypeStr=Inherit: Inherit via back propagation  FilterDenConstantOutMin=[]  FilterDenConstantOutMax=[]  PCopyOutDataTypeStr=Inherit: Inherit via back propagation  PCopyOutMin=[]  PCopyOutMax=[]  NCopyOutDataTypeStr=Inherit: Inherit via back propagation  NCopyOutMin=[]  NCopyOutMax=[]  IntegratorContinuousStateAttributes=''  IntegratorStateMustResolveToSignalObject=off  IntegratorRTWStateStorageClass=Auto  FilterContinuousStateAttributes=''  FilterStateMustResolveToSignalObject=off  FilterRTWStateStorageClass=Auto  ParallelPVariant=InternalParameters  IdealPVariant=Disabled  IVariant=InternalParameters  DVariant=InternalParameters  IntegratorVariant=Continuous  SatVariant=Disabled  AWVariant=Passthrough  PCopyVariant=Disabled  TRVariant=Disabled  FdbkBlocksVariant=Forward  IdealPFdbkVariant=Disabled  SatFdbkVariant=Disabled  DerivativeFilterVariant=ContFilter  NVariant=InternalParameters  NCopyVariant=Disabled  FilterICVariant=InternalICsFilter  IntegratorICVariant=InternalICs  ExternalResetVariant=Disabled  TRSumVariant=Passthrough  SumFdbkVariant=Disabled  SumVariant=Sum_PID  TsampFilterVariant=InternalTs  TsampNgainVariant=Passthrough  TsampIntegralVariant=Passthrough  ExternalSaturationOutDataTypeStr=Inherit: Same as second input
  PID Controller3 : slpidlib/PID Controller  Controller=PID  Form=Parallel  TimeDomain=Continuous-time  UseExternalTs=off  SampleTime=-1  IntegratorMethod=Forward Euler  FilterMethod=Forward Euler  ControllerParametersSource=internal  P=0.5  I=0  UseKiTs=off  D=0  N=100  UseFilter=on  TunerSelectOption=Transfer Function Based (PID Tuner App)  InitialConditionSource=internal  InitialConditionForIntegrator=0  InitialConditionForFilter=0  DifferentiatorICPrevScaledInput=0  ExternalReset=none  TrackingMode=off  Kt=1  LimitOutput=on  SatLimitsSource=internal  UpperSaturationLimit=1  LowerSaturationLimit=-1  LinearizeAsGain=on  AntiWindupMode=none  Kb=1  LimitIntegrator=off  UpperIntegratorSaturationLimit=inf  LowerIntegratorSaturationLimit=-inf  POutMin=[]  POutMax=[]  IOutMin=[]  IOutMax=[]  DOutMin=[]  DOutMax=[]  NOutMin=[]  NOutMax=[]  SumOutMin=[]  SumOutMax=[]  SaturationOutMin=[]  SaturationOutMax=[]  PParamMin=[]  PParamMax=[]  IParamMin=[]  IParamMax=[]  DParamMin=[]  DParamMax=[]  NParamMin=[]  NParamMax=[]  KbParamMin=[]  KbParamMax=[]  KtParamMin=[]  KtParamMax=[]  KbOutMin=[]  KbOutMax=[]  KtOutMin=[]  KtOutMax=[]  IntegratorOutMin=[]  IntegratorOutMax=[]  FilterOutMin=[]  FilterOutMax=[]  SumI1OutMin=[]  SumI1OutMax=[]  SumI2OutMin=[]  SumI2OutMax=[]  SumI3OutMin=[]  SumI3OutMax=[]  SumI4OutMin=[]  SumI4OutMax=[]  SumDOutMin=[]  SumDOutMax=[]  DifferentiatorOutMin=[]  DifferentiatorOutMax=[]  FilterDiffOutCoefMin=[]  FilterDiffOutCoefMax=[]  ReciprocalOutMin=[]  ReciprocalOutMax=[]  SumDenOutMin=[]  SumDenOutMax=[]  SumNumOutMin=[]  SumNumOutMax=[]  DivideOutMin=[]  DivideOutMax=[]  UdiffTsProdOutMin=[]  UdiffTsProdOutMax=[]  NTsProdOutMin=[]  NTsProdOutMax=[]  UintegralTsProdOutMin=[]  UintegralTsProdOutMax=[]  UngainTsProdOutMin=[]  UngainTsProdOutMax=[]  ClampingZeroOutDataTypeStr=Inherit: Inherit via back propagation  ClampingZeroOutMin=[]  ClampingZeroOutMax=[]  FilterDenConstantOutDataTypeStr=Inherit: Inherit via back propagation  FilterDenConstantOutMin=[]  FilterDenConstantOutMax=[]  PCopyOutDataTypeStr=Inherit: Inherit via back propagation  PCopyOutMin=[]  PCopyOutMax=[]  NCopyOutDataTypeStr=Inherit: Inherit via back propagation  NCopyOutMin=[]  NCopyOutMax=[]  IntegratorContinuousStateAttributes=''  IntegratorStateMustResolveToSignalObject=off  IntegratorRTWStateStorageClass=Auto  FilterContinuousStateAttributes=''  FilterStateMustResolveToSignalObject=off  FilterRTWStateStorageClass=Auto  ParallelPVariant=InternalParameters  IdealPVariant=Disabled  IVariant=InternalParameters  DVariant=InternalParameters  IntegratorVariant=Continuous  SatVariant=Enabled  AWVariant=Passthrough  PCopyVariant=Disabled  TRVariant=Disabled  FdbkBlocksVariant=Forward  IdealPFdbkVariant=Disabled  SatFdbkVariant=Disabled  DerivativeFilterVariant=ContFilter  NVariant=InternalParameters  NCopyVariant=Disabled  FilterICVariant=InternalICsFilter  IntegratorICVariant=InternalICs  ExternalResetVariant=Disabled  TRSumVariant=Passthrough  SumFdbkVariant=Disabled  SumVariant=Sum_PID  TsampFilterVariant=InternalTs  TsampNgainVariant=Passthrough  TsampIntegralVariant=Passthrough  ExternalSaturationOutDataTypeStr=Inherit: Same as second input
  tao_X : Outport
  wires:
  PID Controller/1 -> tao_X/1  "tao_X"
  Add4/1 -> PID Controller/1
  PID Controller3/1 -> Add4/2  "ud"
  dx/1 -> PID Controller3/1
  u/1 -> Add4/1  "u"

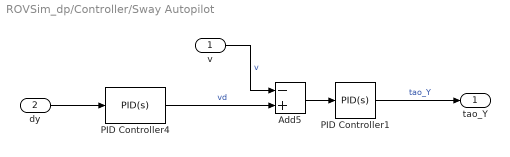
== system ROVSim_dp/Controller/Sway Autopilot ==
  v : Inport
  dy : Inport  Port=2
  Add5 : Sum  Inputs=-+
  PID Controller1 : slpidlib/PID Controller  Controller=PID  Form=Parallel  TimeDomain=Continuous-time  UseExternalTs=off  SampleTime=-1  IntegratorMethod=Forward Euler  FilterMethod=Forward Euler  ControllerParametersSource=internal  P=20  I=0  UseKiTs=off  D=0  N=100  UseFilter=on  TunerSelectOption=Transfer Function Based (PID Tuner App)  InitialConditionSource=internal  InitialConditionForIntegrator=0  InitialConditionForFilter=0  DifferentiatorICPrevScaledInput=0  ExternalReset=none  TrackingMode=off  Kt=1  LimitOutput=off  SatLimitsSource=internal  UpperSaturationLimit=inf  LowerSaturationLimit=-inf  LinearizeAsGain=on  AntiWindupMode=none  Kb=1  LimitIntegrator=off  UpperIntegratorSaturationLimit=inf  LowerIntegratorSaturationLimit=-inf  POutMin=[]  POutMax=[]  IOutMin=[]  IOutMax=[]  DOutMin=[]  DOutMax=[]  NOutMin=[]  NOutMax=[]  SumOutMin=[]  SumOutMax=[]  SaturationOutMin=[]  SaturationOutMax=[]  PParamMin=[]  PParamMax=[]  IParamMin=[]  IParamMax=[]  DParamMin=[]  DParamMax=[]  NParamMin=[]  NParamMax=[]  KbParamMin=[]  KbParamMax=[]  KtParamMin=[]  KtParamMax=[]  KbOutMin=[]  KbOutMax=[]  KtOutMin=[]  KtOutMax=[]  IntegratorOutMin=[]  IntegratorOutMax=[]  FilterOutMin=[]  FilterOutMax=[]  SumI1OutMin=[]  SumI1OutMax=[]  SumI2OutMin=[]  SumI2OutMax=[]  SumI3OutMin=[]  SumI3OutMax=[]  SumI4OutMin=[]  SumI4OutMax=[]  SumDOutMin=[]  SumDOutMax=[]  DifferentiatorOutMin=[]  DifferentiatorOutMax=[]  FilterDiffOutCoefMin=[]  FilterDiffOutCoefMax=[]  ReciprocalOutMin=[]  ReciprocalOutMax=[]  SumDenOutMin=[]  SumDenOutMax=[]  SumNumOutMin=[]  SumNumOutMax=[]  DivideOutMin=[]  DivideOutMax=[]  UdiffTsProdOutMin=[]  UdiffTsProdOutMax=[]  NTsProdOutMin=[]  NTsProdOutMax=[]  UintegralTsProdOutMin=[]  UintegralTsProdOutMax=[]  UngainTsProdOutMin=[]  UngainTsProdOutMax=[]  ClampingZeroOutDataTypeStr=Inherit: Inherit via back propagation  ClampingZeroOutMin=[]  ClampingZeroOutMax=[]  FilterDenConstantOutDataTypeStr=Inherit: Inherit via back propagation  FilterDenConstantOutMin=[]  FilterDenConstantOutMax=[]  PCopyOutDataTypeStr=Inherit: Inherit via back propagation  PCopyOutMin=[]  PCopyOutMax=[]  NCopyOutDataTypeStr=Inherit: Inherit via back propagation  NCopyOutMin=[]  NCopyOutMax=[]  IntegratorContinuousStateAttributes=''  IntegratorStateMustResolveToSignalObject=off  IntegratorRTWStateStorageClass=Auto  FilterContinuousStateAttributes=''  FilterStateMustResolveToSignalObject=off  FilterRTWStateStorageClass=Auto  ParallelPVariant=InternalParameters  IdealPVariant=Disabled  IVariant=InternalParameters  DVariant=InternalParameters  IntegratorVariant=Continuous  SatVariant=Disabled  AWVariant=Passthrough  PCopyVariant=Disabled  TRVariant=Disabled  FdbkBlocksVariant=Forward  IdealPFdbkVariant=Disabled  SatFdbkVariant=Disabled  DerivativeFilterVariant=ContFilter  NVariant=InternalParameters  NCopyVariant=Disabled  FilterICVariant=InternalICsFilter  IntegratorICVariant=InternalICs  ExternalResetVariant=Disabled  TRSumVariant=Passthrough  SumFdbkVariant=Disabled  SumVariant=Sum_PID  TsampFilterVariant=InternalTs  TsampNgainVariant=Passthrough  TsampIntegralVariant=Passthrough  ExternalSaturationOutDataTypeStr=Inherit: Same as second input
  PID Controller4 : slpidlib/PID Controller  Controller=PID  Form=Parallel  TimeDomain=Continuous-time  UseExternalTs=off  SampleTime=-1  IntegratorMethod=Forward Euler  FilterMethod=Forward Euler  ControllerParametersSource=internal  P=0.5  I=0  UseKiTs=off  D=0  N=100  UseFilter=on  TunerSelectOption=Transfer Function Based (PID Tuner App)  InitialConditionSource=internal  InitialConditionForIntegrator=0  InitialConditionForFilter=0  DifferentiatorICPrevScaledInput=0  ExternalReset=none  TrackingMode=off  Kt=1  LimitOutput=on  SatLimitsSource=internal  UpperSaturationLimit=1  LowerSaturationLimit=-1  LinearizeAsGain=on  AntiWindupMode=none  Kb=1  LimitIntegrator=off  UpperIntegratorSaturationLimit=inf  LowerIntegratorSaturationLimit=-inf  POutMin=[]  POutMax=[]  IOutMin=[]  IOutMax=[]  DOutMin=[]  DOutMax=[]  NOutMin=[]  NOutMax=[]  SumOutMin=[]  SumOutMax=[]  SaturationOutMin=[]  SaturationOutMax=[]  PParamMin=[]  PParamMax=[]  IParamMin=[]  IParamMax=[]  DParamMin=[]  DParamMax=[]  NParamMin=[]  NParamMax=[]  KbParamMin=[]  KbParamMax=[]  KtParamMin=[]  KtParamMax=[]  KbOutMin=[]  KbOutMax=[]  KtOutMin=[]  KtOutMax=[]  IntegratorOutMin=[]  IntegratorOutMax=[]  FilterOutMin=[]  FilterOutMax=[]  SumI1OutMin=[]  SumI1OutMax=[]  SumI2OutMin=[]  SumI2OutMax=[]  SumI3OutMin=[]  SumI3OutMax=[]  SumI4OutMin=[]  SumI4OutMax=[]  SumDOutMin=[]  SumDOutMax=[]  DifferentiatorOutMin=[]  DifferentiatorOutMax=[]  FilterDiffOutCoefMin=[]  FilterDiffOutCoefMax=[]  ReciprocalOutMin=[]  ReciprocalOutMax=[]  SumDenOutMin=[]  SumDenOutMax=[]  SumNumOutMin=[]  SumNumOutMax=[]  DivideOutMin=[]  DivideOutMax=[]  UdiffTsProdOutMin=[]  UdiffTsProdOutMax=[]  NTsProdOutMin=[]  NTsProdOutMax=[]  UintegralTsProdOutMin=[]  UintegralTsProdOutMax=[]  UngainTsProdOutMin=[]  UngainTsProdOutMax=[]  ClampingZeroOutDataTypeStr=Inherit: Inherit via back propagation  ClampingZeroOutMin=[]  ClampingZeroOutMax=[]  FilterDenConstantOutDataTypeStr=Inherit: Inherit via back propagation  FilterDenConstantOutMin=[]  FilterDenConstantOutMax=[]  PCopyOutDataTypeStr=Inherit: Inherit via back propagation  PCopyOutMin=[]  PCopyOutMax=[]  NCopyOutDataTypeStr=Inherit: Inherit via back propagation  NCopyOutMin=[]  NCopyOutMax=[]  IntegratorContinuousStateAttributes=''  IntegratorStateMustResolveToSignalObject=off  IntegratorRTWStateStorageClass=Auto  FilterContinuousStateAttributes=''  FilterStateMustResolveToSignalObject=off  FilterRTWStateStorageClass=Auto  ParallelPVariant=InternalParameters  IdealPVariant=Disabled  IVariant=InternalParameters  DVariant=InternalParameters  IntegratorVariant=Continuous  SatVariant=Enabled  AWVariant=Passthrough  PCopyVariant=Disabled  TRVariant=Disabled  FdbkBlocksVariant=Forward  IdealPFdbkVariant=Disabled  SatFdbkVariant=Disabled  DerivativeFilterVariant=ContFilter  NVariant=InternalParameters  NCopyVariant=Disabled  FilterICVariant=InternalICsFilter  IntegratorICVariant=InternalICs  ExternalResetVariant=Disabled  TRSumVariant=Passthrough  SumFdbkVariant=Disabled  SumVariant=Sum_PID  TsampFilterVariant=InternalTs  TsampNgainVariant=Passthrough  TsampIntegralVariant=Passthrough  ExternalSaturationOutDataTypeStr=Inherit: Same as second input
  tao_Y : Outport
  wires:
  PID Controller1/1 -> tao_Y/1  "tao_Y"
  PID Controller4/1 -> Add5/2  "vd"
  Add5/1 -> PID Controller1/1
  dy/1 -> PID Controller4/1
  v/1 -> Add5/1  "v"

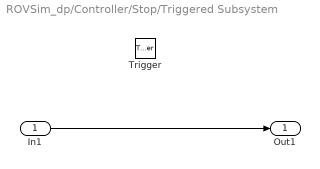
== system ROVSim_dp/Controller/Stop/Triggered Subsystem ==
  In1 : Inport
  Trigger : TriggerPort  TriggerType=falling  VariantControl=Variant
  Out1 : Outport  InitialOutput=1000
  wires:
  In1/1 -> Out1/1

== system ROVSim_dp/Controller/Stop/Triggered Subsystem1 ==
  Trigger : TriggerPort  VariantControl=Variant
  Constant : Constant
  Stop Simulation : Stop
  wires:
  Constant/1 -> Stop Simulation/1

== matlab function ROVSim_dp/Kinematics/MATLAB Function ==
  data: flowDir input; flowu output; flowVel input; psi input; flowv output
function [flowu,flowv] = fcn(flowDir,flowVel,psi)
dAngle = flowDir - psi;
if dAngle > 2*pi
    dAngle = dAngle-2*pi;
elseif dAngle<0
    dAngle = dAngle+2*pi;
end
flowu = flowVel*cos(dAngle);
flowv = flowVel*sin(dAngle);

== matlab function ROVSim_dp/Thrusters/MATLAB Function ==
  data: u input; y output; up input; low input
function y = fcn(u,up,low) % 过滤掉在low和up之间的信号（这些信号可能不是我们所希望看到的，比如干扰）
y = u;
for i=1:8
    if y(i) < up && y(i) >low
        y(i) = 0;
    end
end
end

== matlab function ROVSim_dp/Controller/MATLAB Function ==
  data: dp input; Yaw input; dx output; dy output; dz output
function [dx,dy,dz] = fcn(dp,Yaw)
psi = Yaw/180*pi;
y = [cos(psi) sin(psi); -sin(psi) cos(psi)]*dp(1:2);
dx = y(1);
dy = y(2);
dz = dp(3);
